simulink model "Trajektorien_test"  (R2020a)
settings: Solver=ode45  StartTime=0.0  StopTime=3.5  FixedStep=0.01  RelTol=1e-10
settings Model: Creator=Frederik  LastModifiedBy=Frederik

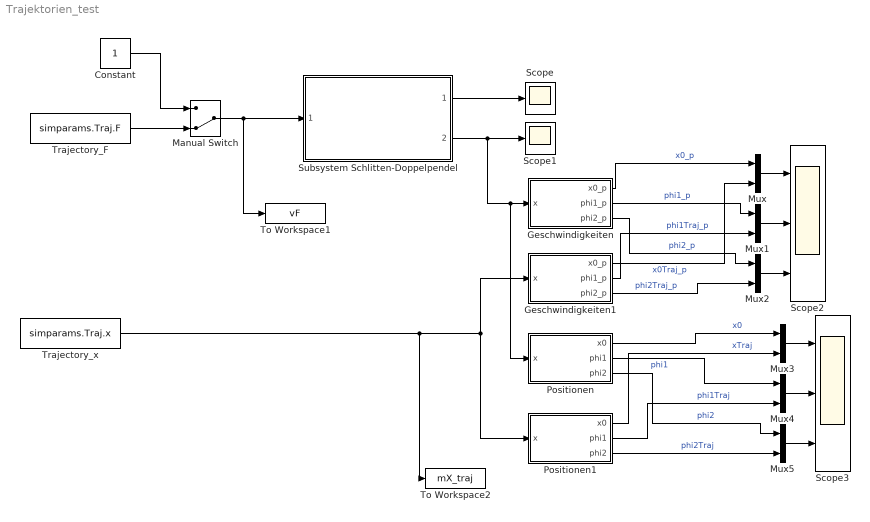
== system Trajektorien_test ==
  Constant : Constant
  Geschwindigkeiten : Subsystem
  Geschwindigkeiten1 : Subsystem
  Manual Switch : ManualSwitch  CurrentSetting=0
  Mux{,1..5} (6 alike) : Mux  Inputs=2
  Positionen : Subsystem
  Positionen1 : Subsystem
  Scope : Scope
  Scope1 : Scope
  Scope2 : Scope  NumInputPorts=3
  Scope3 : Scope  NumInputPorts=3
  Subsystem Schlitten-Doppelpendel : Subsystem  ReferencedSubsystem=SchlittenPendel  params=simparams.gesamtmodell.schlittenpendel
  To Workspace1 : ToWorkspace  VariableName=vF  SaveFormat=Timeseries  SampleTime=-1
  To Workspace2 : ToWorkspace  VariableName=mX_traj  SaveFormat=Timeseries  SampleTime=-1
  Trajectory_F : FromWorkspace  VariableName=simparams.Traj.F  Interpolate=off  OutputAfterFinalValue=Setting to zero
  Trajectory_x : FromWorkspace  VariableName=simparams.Traj.x  Interpolate=off  OutputAfterFinalValue=Setting to zero
  wires:
  Manual Switch/1 -> To Workspace1/1, Subsystem Schlitten-Doppelpendel/1
  Subsystem Schlitten-Doppelpendel/1 -> Scope/1
  Trajectory_F/1 -> Manual Switch/2
  Constant/1 -> Manual Switch/1
  Subsystem Schlitten-Doppelpendel/2 -> Positionen/1(x), Geschwindigkeiten/1(x), Scope1/1
  Geschwindigkeiten/1(x0_p) -> Mux/1  "x0_p"
  Geschwindigkeiten/2(phi1_p) -> Mux1/1  "phi1_p"
  Geschwindigkeiten/3(phi2_p) -> Mux2/1  "phi2_p"
  Trajectory_x/1 -> To Workspace2/1, Positionen1/1(x), Geschwindigkeiten1/1(x)
  Geschwindigkeiten1/1(x0_p) -> Mux/2  "x0Traj_p"
  Geschwindigkeiten1/2(phi1_p) -> Mux1/2  "phi1Traj_p"
  Geschwindigkeiten1/3(phi2_p) -> Mux2/2  "phi2Traj_p"
  Mux2/1 -> Scope2/3
  Mux1/1 -> Scope2/2
  Mux/1 -> Scope2/1
  Positionen/3(phi2) -> Mux5/1  "phi2"
  Mux4/1 -> Scope3/2
  Mux5/1 -> Scope3/3
  Mux3/1 -> Scope3/1
  Positionen/1(x0) -> Mux3/1  "x0"
  Positionen1/1(x0) -> Mux3/2  "xTraj"
  Positionen1/2(phi1) -> Mux4/2  "phi1Traj"
  Positionen1/3(phi2) -> Mux5/2  "phi2Traj"
  Positionen/2(phi1) -> Mux4/1  "phi1"

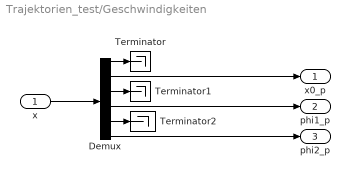
== system Trajektorien_test/Geschwindigkeiten ==
  x : Inport
  Demux : Demux  Outputs=6
  Terminator : Terminator
  Terminator1 : Terminator
  Terminator2 : Terminator
  x0_p : Outport
  phi1_p : Outport  Port=2
  phi2_p : Outport  Port=3
  wires:
  Demux/4 -> phi1_p/1
  Demux/2 -> x0_p/1
  Demux/5 -> Terminator2/1
  x/1 -> Demux/1
  Demux/3 -> Terminator1/1
  Demux/1 -> Terminator/1
  Demux/6 -> phi2_p/1

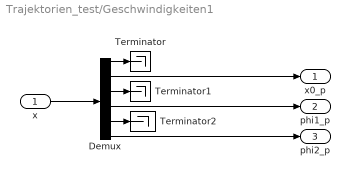
== system Trajektorien_test/Geschwindigkeiten1 ==
  x : Inport
  Demux : Demux  Outputs=6
  Terminator : Terminator
  Terminator1 : Terminator
  Terminator2 : Terminator
  x0_p : Outport
  phi1_p : Outport  Port=2
  phi2_p : Outport  Port=3
  wires:
  Demux/4 -> phi1_p/1
  Demux/2 -> x0_p/1
  Demux/5 -> Terminator2/1
  x/1 -> Demux/1
  Demux/3 -> Terminator1/1
  Demux/1 -> Terminator/1
  Demux/6 -> phi2_p/1

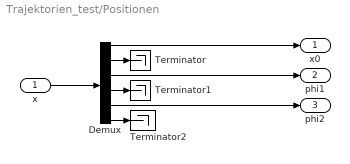
== system Trajektorien_test/Positionen ==
  x : Inport
  Demux : Demux  Outputs=6
  Terminator : Terminator
  Terminator1 : Terminator
  Terminator2 : Terminator
  x0 : Outport
  phi1 : Outport  Port=2
  phi2 : Outport  Port=3
  wires:
  Demux/3 -> phi1/1
  Demux/1 -> x0/1
  x/1 -> Demux/1
  Demux/5 -> phi2/1
  Demux/2 -> Terminator/1
  Demux/4 -> Terminator1/1
  Demux/6 -> Terminator2/1

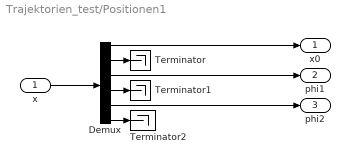
== system Trajektorien_test/Positionen1 ==
  x : Inport
  Demux : Demux  Outputs=6
  Terminator : Terminator
  Terminator1 : Terminator
  Terminator2 : Terminator
  x0 : Outport
  phi1 : Outport  Port=2
  phi2 : Outport  Port=3
  wires:
  Demux/3 -> phi1/1
  Demux/1 -> x0/1
  x/1 -> Demux/1
  Demux/5 -> phi2/1
  Demux/2 -> Terminator/1
  Demux/4 -> Terminator1/1
  Demux/6 -> Terminator2/1
